simulink model "TrabControle"  (R2018b)
settings: Solver=VariableStepAuto  StartTime=0.0  StopTime=100  RelTol=1e-3
libraries: simulink x28
settings Model: Creator=Azeli  LastModifiedBy=Azeli

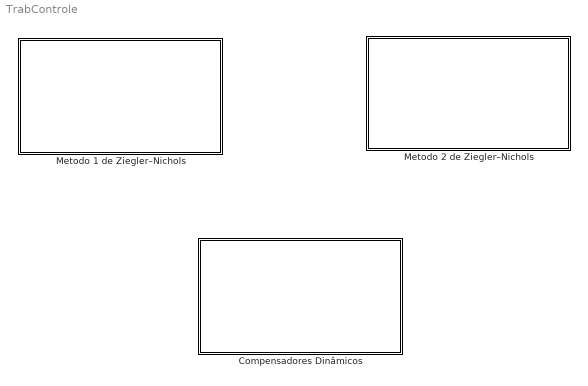
== system TrabControle ==
  Compensadores Dinâmicos : Subsystem
  "Metodo 1 de Ziegler–Nichols " : Subsystem
  "Metodo 2 de Ziegler–Nichols " : Subsystem

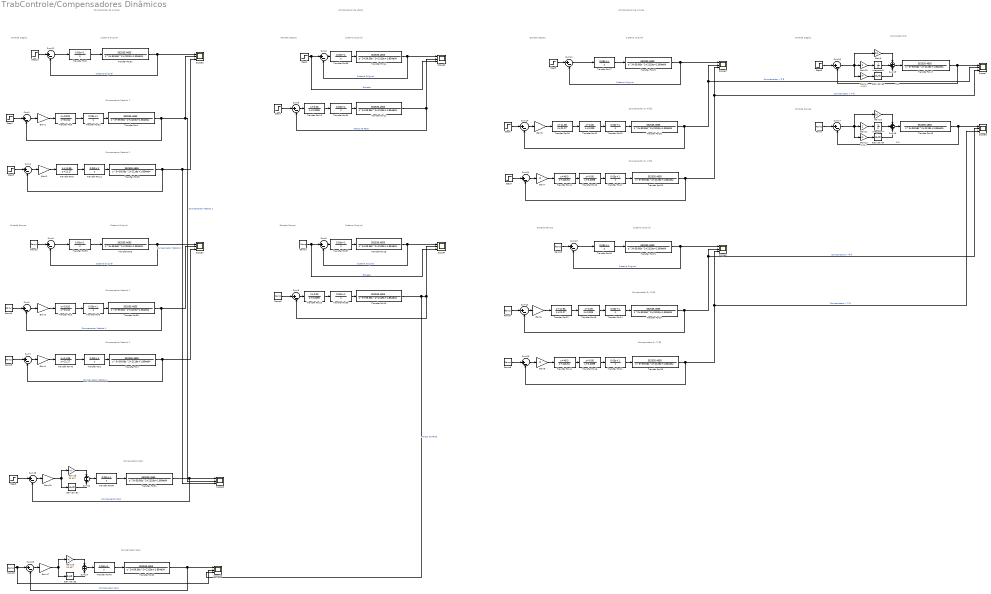
== system TrabControle/Compensadores Dinâmicos ==
  note: Compensador de Avanço
  note: Sistema Original
  note: Compensador Método 1
  note: Compensador Método 2
  note: Sistema Original
  note: Entrada Degrau
  note: Entrada Rampa
  note: Compensador de Atraso
  note: Sistema Original
  note: Sistema Original
  note: Entrada Rampa
  note: Entrada Degrau
  note: Compensador de Avanço
  note: Entrada Degrau
  note: Sistema Original
  note: Entrada Rampa
  note: Sistema Original
  note: Compensador Método 1
  note: Compensador Método 2
  note: Compensador $γ ≠ β$
  note: Compensador $γ = β$
  note: Compensador $γ ≠ β$
  note: Compensador $γ = β$
  note: Controlador PID
  note: Entrada Degrau
  note: Entrada Rampa
  note: Compensador Zero
  note: Compensador Zero
  Derivative{1..4} (4 alike) : Derivative
  Gain1 : Gain  Gain=1.6644
  Gain10 : Gain  Gain=0.1
  Gain11 : Gain  Gain=2
  Gain12 : Gain  Gain=0.004
  Gain13 : Gain  Gain=2
  Gain14 : Gain  Gain=0.004
  Gain15 : Gain  Gain=0.0290
  Gain16 : Gain  Gain=55.897
  Gain17 : Gain  Gain=0.0290
  Gain18 : Gain  Gain=55.897
  Gain{2,4..6} (4 alike) : Gain  Gain=1.3668
  Gain3 : Gain  Gain=1.6644
  Gain7 : Gain  Gain=8
  Gain8 : Gain  Gain=8
  Gain9 : Gain  Gain=0.1
  Integrator3 : Integrator
  Integrator4 : Integrator
  Ramp{,1..9} (10 alike) : simulink/Sources/Ramp  slope=1  start=0  InitialOutput=0
  Scope{1..10} (10 alike) : Scope  NumInputPorts=3
  Step{1..10} (10 alike) : Step  Time=0  After=10  SampleTime=0
  Sum{1..15,17..18,20..21,23} (20 alike) : Sum  Inputs=|+-
  Sum16 : Sum  Inputs=+++
  Sum19 : Sum  Inputs=+++
  Sum22 : Sum
  Sum24 : Sum
  Transfer Fcn{1,6,8,11,17,20..21,24,27,30,32,34..37,39,49..50} (18 alike) : TransferFcn  Numerator=[0.03 1]  Denominator=[1 0]
  Transfer Fcn{4..5,7,10,12,14,16,19,23,25..26,28..29,31,33,38,47..48,51..52} (20 alike) : TransferFcn  Numerator=[352535.4655]  Denominator=[1 59.56 2119 1.854e04]
  Transfer Fcn13 : TransferFcn  Numerator=[1 0.05]  Denominator=[1 0.0095]
  Transfer Fcn15 : TransferFcn  Numerator=[1 0.05]  Denominator=[1 0.0095]
  Transfer Fcn{9,18,22,40} (4 alike) : TransferFcn  Numerator=[1 11.96]  Denominator=[1 21.27]
  Transfer Fcn2 : TransferFcn  Numerator=[1 19.81]  Denominator=[1 31.54]
  Transfer Fcn3 : TransferFcn  Numerator=[1 19.81]  Denominator=[1 31.54]
  Transfer Fcn41 : TransferFcn  Numerator=[1 48.3]  Denominator=[1 246.91]
  Transfer Fcn42 : TransferFcn  Numerator=[1 0.06]  Denominator=[1 0.005]
  Transfer Fcn43 : TransferFcn  Numerator=[1 0.05]  Denominator=[1 0.0098]
  Transfer Fcn44 : TransferFcn  Numerator=[1 48.3]  Denominator=[1 246.91]
  Transfer Fcn45 : TransferFcn  Numerator=[1 0.06]  Denominator=[1 0.005]
  Transfer Fcn46 : TransferFcn  Numerator=[1 0.05]  Denominator=[1 0.0098]
  wires:
  Transfer Fcn4/1 -> Sum1/2, Scope9/2, Scope2/2  "Compensador Método 1"
  Step2/1 -> Sum1/1
  Step10/1 -> Sum21/1
  Sum21/1 -> Transfer Fcn8/1
  Transfer Fcn3/1 -> Transfer Fcn32/1
  Gain1/1 -> Transfer Fcn3/1
  Sum1/1 -> Gain1/1
  Transfer Fcn31/1 -> Sum21/2, Scope2/1  "Sistema Original"
  Transfer Fcn33/1 -> Sum4/2, Scope9/3, Scope2/3  "Compensador Método 2"
  Step4/1 -> Sum5/1
  Transfer Fcn12/1 -> Scope3/2, Sum5/2  "Atraso de Fase"
  Sum5/1 -> Transfer Fcn13/1
  Transfer Fcn14/1 -> Scope3/1, Sum6/2  "Sistema Original"
  Step1/1 -> Scope3/3, Sum6/1  "Entrada"
  Ramp2/1 -> Sum2/1
  Ramp5/1 -> Sum7/1
  Ramp6/1 -> Sum8/1
  Transfer Fcn8/1 -> Transfer Fcn31/1
  Transfer Fcn32/1 -> Transfer Fcn4/1
  Step3/1 -> Sum4/1
  Transfer Fcn9/1 -> Transfer Fcn11/1
  Sum4/1 -> Gain2/1
  Transfer Fcn11/1 -> Transfer Fcn33/1
  Gain2/1 -> Transfer Fcn9/1
  Transfer Fcn13/1 -> Transfer Fcn34/1
  Transfer Fcn34/1 -> Transfer Fcn12/1
  Sum6/1 -> Transfer Fcn35/1
  Transfer Fcn35/1 -> Transfer Fcn14/1
  Sum9/1 -> Transfer Fcn37/1
  Transfer Fcn37/1 -> Transfer Fcn16/1
  Sum8/1 -> Transfer Fcn15/1
  Ramp7/1 -> Scope4/3, Sum9/1  "Entrada"
  Transfer Fcn36/1 -> Transfer Fcn10/1
  Transfer Fcn15/1 -> Transfer Fcn36/1
  Transfer Fcn16/1 -> Scope4/1, Sum9/2  "Sistema Original"
  Transfer Fcn10/1 -> Scope10/3, Scope4/2, Sum8/2  "Atraso de Fase"
  Transfer Fcn1/1 -> Transfer Fcn7/1
  Transfer Fcn40/1 -> Transfer Fcn1/1
  Transfer Fcn6/1 -> Transfer Fcn38/1
  Transfer Fcn39/1 -> Transfer Fcn5/1
  Transfer Fcn5/1 -> Sum3/2, Scope1/1  "Sistema Original"
  Transfer Fcn2/1 -> Transfer Fcn6/1
  Gain3/1 -> Transfer Fcn2/1
  Sum2/1 -> Gain3/1
  Transfer Fcn7/1 -> Sum7/2, Scope1/3  "Compensador Método 2"
  Sum7/1 -> Gain4/1
  Sum3/1 -> Transfer Fcn39/1
  Transfer Fcn38/1 -> Sum2/2, Scope1/2  "Compensador Método 1"
  Ramp1/1 -> Sum3/1
  Gain7/1 -> Transfer Fcn41/1
  Transfer Fcn17/1 -> Transfer Fcn25/1
  Transfer Fcn20/1 -> Transfer Fcn26/1
  Step6/1 -> Sum10/1
  Transfer Fcn27/1 -> Transfer Fcn19/1
  Transfer Fcn19/1 -> Sum11/2, Scope5/1  "Sistema Original"
  Step7/1 -> Sum14/1
  Transfer Fcn25/1 -> Sum14/2, Scope7/3, Scope5/3  "Compensador γ = β"
  Sum14/1 -> Gain7/1
  Sum11/1 -> Transfer Fcn27/1
  Transfer Fcn26/1 -> Sum10/2, Scope5/2, Scope7/2  "Compensador γ ≠ β"
  Step5/1 -> Sum11/1
  Transfer Fcn42/1 -> Transfer Fcn20/1
  Transfer Fcn18/1 -> Transfer Fcn42/1
  Transfer Fcn41/1 -> Transfer Fcn43/1
  Transfer Fcn43/1 -> Transfer Fcn17/1
  Transfer Fcn44/1 -> Transfer Fcn46/1
  Transfer Fcn46/1 -> Transfer Fcn21/1
  Sum13/1 -> Transfer Fcn30/1
  Transfer Fcn29/1 -> Sum12/2, Scope8/2, Scope6/2  "Compensador γ ≠ β"
  Ramp4/1 -> Sum12/1
  Sum12/1 -> Gain6/1
  Transfer Fcn30/1 -> Transfer Fcn23/1
  Sum15/1 -> Gain8/1
  Transfer Fcn24/1 -> Transfer Fcn29/1
  Transfer Fcn21/1 -> Transfer Fcn28/1
  Transfer Fcn45/1 -> Transfer Fcn24/1
  Transfer Fcn28/1 -> Sum15/2, Scope8/3, Scope6/3  "Compensador γ = β"
  Ramp8/1 -> Sum15/1
  Gain8/1 -> Transfer Fcn44/1
  Transfer Fcn23/1 -> Sum13/2, Scope6/1  "Sistema Original"
  Ramp3/1 -> Sum13/1
  Gain4/1 -> Transfer Fcn40/1
  Gain5/1 -> Transfer Fcn18/1
  Sum10/1 -> Gain5/1
  Transfer Fcn22/1 -> Transfer Fcn45/1
  Gain6/1 -> Transfer Fcn22/1
  Gain9/1 -> Sum19/1
  Gain11/1 -> Integrator4/1
  Sum19/1 -> Transfer Fcn47/1
  Sum20/1 -> Gain9/1, Gain14/1, Gain13/1
  Integrator4/1 -> Sum16/2
  Gain13/1 -> Integrator3/1
  Derivative3/1 -> Sum19/3
  Integrator3/1 -> Sum19/2
  Gain10/1 -> Sum16/1
  Transfer Fcn47/1 -> Scope7/1, Sum20/2  "PID"
  Sum17/1 -> Gain10/1, Gain12/1, Gain11/1
  Step8/1 -> Sum20/1
  Transfer Fcn48/1 -> Scope8/1, Sum17/2  "PID"
  Sum16/1 -> Transfer Fcn48/1
  Gain14/1 -> Derivative3/1
  Ramp/1 -> Sum17/1
  Derivative4/1 -> Sum16/3
  Gain12/1 -> Derivative4/1
  Transfer Fcn50/1 -> Transfer Fcn51/1
  Sum18/1 -> Gain15/1
  Gain15/1 -> Derivative1/1, Gain16/1
  Sum22/1 -> Transfer Fcn50/1
  Step9/1 -> Sum18/1
  Transfer Fcn51/1 -> Scope9/1, Sum18/2  "Compensador Zero"
  Gain16/1 -> Sum22/1
  Derivative1/1 -> Sum22/2
  Transfer Fcn52/1 -> Scope10/1, Sum23/2  "Compensador Zero"
  Ramp9/1 -> Scope10/2, Sum23/1
  Sum23/1 -> Gain17/1
  Transfer Fcn49/1 -> Transfer Fcn52/1
  Gain18/1 -> Sum24/1
  Sum24/1 -> Transfer Fcn49/1
  Gain17/1 -> Derivative2/1, Gain18/1
  Derivative2/1 -> Sum24/2

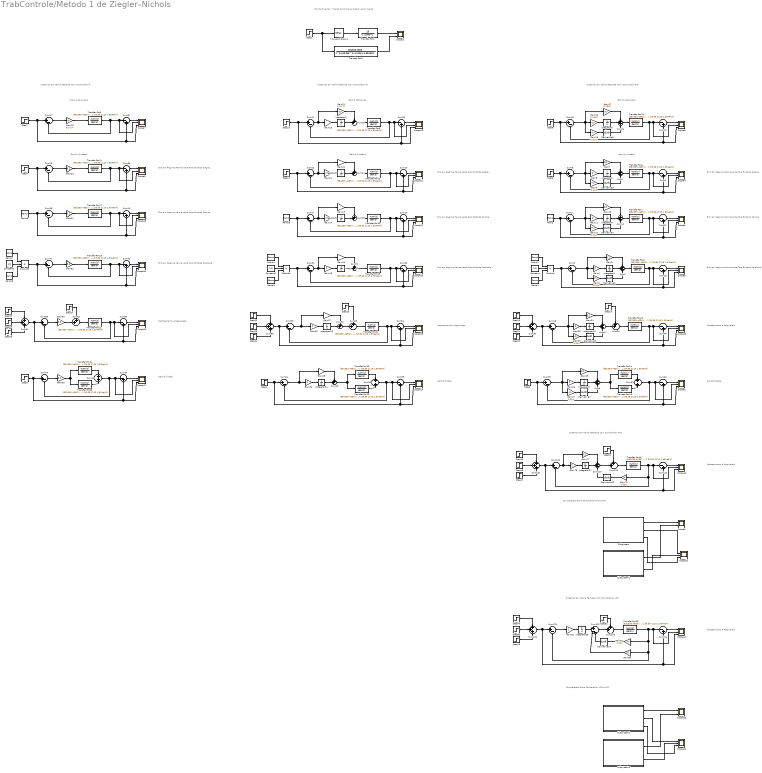
== system TrabControle/Metodo 1 de Ziegler–Nichols  ==
  note: Ganho Calculado
  note: Planta Original x Planta de Primeira Ordem Aproximada
  note: Sistemas em Malha Fechada Com Controlador P
  note: Ganho Ajustado
  note: Erro em Regime Permanente Para Entrada Degrau
  note: Erro em Regime Permanente Para Entrada Rampa
  note: Erro em Regime Permanente Para Entrada Parábola
  note: Rastreamento e Regulação
  note: Sensibilidade
  note: Erro em Regime Permanente Para Entrada Degrau
  note: Erro em Regime Permanente Para Entrada Parábola
  note: Sensibilidade
  note: Erro em Regime Permanente Para Entrada Rampa
  note: Rastreamento e Regulação
  note: Ganho Calculado
  note: Sistemas em Malha Fechada Com Controlador PI
  note: Ganho Ajustado
  note: Sensibilidade
  note: Erro em Regime Permanente Para Entrada Degrau
  note: Rastreamento e Regulação
  note: Erro em Regime Permanente Para Entrada Rampa
  note: Erro em Regime Permanente Para Entrada Parábola
  note: Ganho Calculado
  note: Sistemas em Malha Fechada Com Controlador PID
  note: Sistemas em Malha Fechada Com Controlador PI-D
  note: Sistemas em Malha Fechada Com Controlador I-PD
  note: Rastreamento e Regulação
  note: Rastreamento e Regulação
  note: Ganho Ajustado
  note: Comparação Entre Controlador PI-D e PID
  note: Comparação Entre Controlador I-PD e PID
  Constant : Constant  Value=1/2
  Constant1 : Constant  Value=1/2
  Constant2 : Constant  Value=1/2
  Derivative{1,3..7,13..14} (8 alike) : Derivative
  Gain{3,7,10,20,25,31..34,39,77,80} (12 alike) : Gain  Gain=0.1
  Gain{4,8,11,26,35,78,81} (7 alike) : Gain  Gain=2
  Gain{5,9,12,27,36,79,82} (7 alike) : Gain  Gain=0.004
  Gain{13,15,22,29,37} (5 alike) : Gain  Gain=0.06
  Gain{14,24,28,30,38} (5 alike) : Gain
  Gain16 : Gain  Gain=0.2414
  Gain17 : Gain  Gain=0.2897
  Gain18 : Gain  Gain=5.1548
  Gain19 : Gain  Gain=0.0041
  Gain21 : Gain  Gain=0.2173
  Gain23 : Gain  Gain=2.32
  Integrator{1,3..13,27..28} (14 alike) : Integrator
  Product : Product  Inputs=3
  Product1 : Product  Inputs=3
  Product2 : Product  Inputs=3
  Ramp{,1..8} (9 alike) : simulink/Sources/Ramp  slope=1  start=0  InitialOutput=0
  Scope1 : Scope  NumInputPorts=2
  Scope{2,4..22,40..41} (22 alike) : Scope  NumInputPorts=3
  Scope23 : Scope  NumInputPorts=2
  Scope3 : Scope  NumInputPorts=2
  Step1 : Step  Time=0  SampleTime=0
  Step{2,4..11,18,22,26,43..44} (14 alike) : Step  Time=0  After=10  SampleTime=0
  Step{19,23,27,51..52} (5 alike) : Step  Time=8  After=2  SampleTime=0
  Step{20,24,28,47,49} (5 alike) : Step  Time=6  After=5  SampleTime=0
  Step{21,25,29,48,50} (5 alike) : Step  Time=3  After=-10  SampleTime=0
  Subsystem : Subsystem
  Subsystem1 : Subsystem
  Subsystem2 : Subsystem
  Subsystem3 : Subsystem
  Sum{2,6..7,10,16,47,51,56,61,131..132} (11 alike) : Sum  Inputs=+++
  Sum{3,8,11,17..18,20..22,25,27,31,34,39,41,44,48,53,58,120,123} (20 alike) : Sum  Inputs=|+-
  Sum119 : Sum  Inputs=++-
  Sum{9,12..15,19,26,29..30,35,37..38,40,42,45,49,54,59,121,124} (20 alike) : Sum  Inputs=|-+
  Sum122 : Sum  Inputs=|+|--
  Sum{23..24,28,32,43,50,52,55,60,133..134} (11 alike) : Sum  Inputs=++|
  Sum33 : Sum  Inputs=+|+
  Sum36 : Sum  Inputs=+|+
  Sum46 : Sum  Inputs=+|+
  Transfer Fcn1 : TransferFcn  Numerator=[19]  Denominator=[0.1289 1]
  Transfer Fcn{2,5..25,48..49} (24 alike) : TransferFcn  Numerator=[352535.4655]  Denominator=[1 59.56 2119 1.854e04]
  Transport Delay1 : TransportDelay  DelayTime=0.0281
  wires:
  Sum31/1 -> Gain15/1, Gain28/1
  Gain4/1 -> Integrator1/1
  Transfer Fcn1/1 -> Scope1/1
  Ramp3/1 -> Scope12/3, Sum14/2, Sum27/1
  Step9/1 -> Sum38/2, Scope9/3, Sum20/1
  Transfer Fcn48/1 -> Sum120/2, Gain79/1, Scope40/2, Sum121/1
  Transfer Fcn8/1 -> Scope10/2, Sum29/1, Sum21/2
  Transfer Fcn24/1 -> Sum46/1
  Product/1 -> Sum3/1, Sum15/2, Scope6/3
  Sum45/1 -> Scope17/1
  Gain27/1 -> Derivative7/1
  Derivative6/1 -> Sum16/3
  Gain32/1 -> Transfer Fcn18/1
  Transfer Fcn10/1 -> Scope8/2, Sum19/1, Sum18/2
  Sum19/1 -> Scope8/1
  Integrator5/1 -> Sum28/2
  Step7/1 -> Sum37/2, Scope7/3, Sum17/1
  Sum38/1 -> Scope9/1
  Sum56/1 -> Sum54/2, Scope19/3, Sum53/1
  Step1/1 -> Transfer Fcn5/1, Transport Delay1/1
  Ramp5/1 -> Product1/3
  Transfer Fcn21/1 -> Scope19/2, Sum54/1, Sum53/2
  Step11/1 -> Scope11/3, Sum13/2, Sum22/1
  Sum7/1 -> Transfer Fcn6/1
  Derivative3/1 -> Sum7/3
  Gain26/1 -> Integrator9/1
  Gain36/1 -> Derivative5/1
  Step8/1 -> Sum19/2, Scope8/3, Sum18/1
  Transfer Fcn6/1 -> Scope4/2, Sum9/1, Sum8/2
  Transport Delay1/1 -> Transfer Fcn1/1
  Step49/1 -> Sum132/3
  Sum3/1 -> Gain3/1, Gain5/1, Gain4/1
  Derivative4/1 -> Sum10/3
  Ramp1/1 -> Product/1
  Ramp2/1 -> Product/3
  Sum21/1 -> Gain21/1, Gain23/1
  Transfer Fcn5/1 -> Scope1/2
  Step6/1 -> Sum9/2, Scope4/3, Sum8/1
  Sum39/1 -> Gain31/1
  Gain25/1 -> Sum6/1
  Step2/1 -> Sum26/2, Scope2/3, Sum25/1
  Integrator1/1 -> Sum2/2
  Step43/1 -> Sum131/1
  Gain9/1 -> Derivative3/1
  Product2/1 -> Sum42/2, Scope16/3, Sum41/1
  Gain8/1 -> Integrator3/1
  Gain11/1 -> Integrator4/1
  Transfer Fcn7/1 -> Scope5/2, Sum12/1, Sum11/2
  Sum50/1 -> Transfer Fcn20/1
  Integrator6/1 -> Sum16/2
  Sum27/1 -> Gain13/1, Gain14/1
  Sum47/1 -> Sum50/2
  Sum2/1 -> Transfer Fcn2/1
  Integrator12/1 -> Sum47/2
  Gain12/1 -> Derivative4/1
  Transfer Fcn17/1 -> Sum39/2, Scope15/2, Sum40/1
  Step21/1 -> Sum51/2
  Sum16/1 -> Transfer Fcn10/1
  Sum33/1 -> Scope2/2, Sum26/1, Sum25/2
  Sum54/1 -> Scope19/1
  Sum10/1 -> Transfer Fcn7/1
  Sum17/1 -> Gain16/1
  Sum46/1 -> Scope17/2, Sum45/1, Sum44/2
  Step24/1 -> Sum56/3
  Gain17/1 -> Sum16/1
  Gain82/1 -> Derivative14/1
  Gain24/1 -> Integrator8/1
  Transfer Fcn12/1 -> Scope11/2, Sum13/1, Sum22/2
  Sum32/1 -> Transfer Fcn15/1
  Transfer Fcn49/1 -> Sum123/2, Gain80/1, Gain82/1, Scope41/2, Sum124/1
  Sum15/1 -> Scope6/1
  Transfer Fcn20/1 -> Scope18/2, Sum49/1, Sum48/2
  Sum24/1 -> Transfer Fcn12/1
  Sum133/1 -> Transfer Fcn48/1
  Transfer Fcn11/1 -> Sum20/2, Scope9/2, Sum38/1
  Transfer Fcn18/1 -> Sum41/2, Scope16/2, Sum42/1
  Ramp/1 -> Sum12/2, Scope5/3, Sum11/1
  Gain16/1 -> Transfer Fcn9/1
  Sum53/1 -> Gain38/1, Gain37/1
  Gain22/1 -> Sum24/1
  Sum30/1 -> Scope13/1
  Sum22/1 -> Gain22/1, Gain24/1
  Transfer Fcn9/1 -> Sum17/2, Scope7/2, Sum37/1
  Sum25/1 -> Gain25/1, Gain27/1, Gain26/1
  Sum23/1 -> Transfer Fcn8/1
  Gain15/1 -> Sum32/1
  Sum11/1 -> Gain10/1, Gain12/1, Gain11/1
  Step28/1 -> Sum61/3
  Sum37/1 -> Scope7/1
  Transfer Fcn14/1 -> Sum33/1
  Ramp4/1 -> Product1/1
  Transfer Fcn22/1 -> Scope20/2, Sum59/1, Sum58/2
  Ramp6/1 -> Sum40/2, Scope15/3, Sum39/1
  Sum18/1 -> Gain17/1, Gain19/1, Gain18/1
  Gain33/1 -> Transfer Fcn25/1, Transfer Fcn24/1
  Step4/1 -> Sum35/2, Scope14/3, Sum34/1
  Constant1/1 -> Product1/2
  Sum8/1 -> Gain7/1, Gain9/1, Gain8/1
  Step10/1 -> Sum29/2, Scope10/3, Sum21/1
  Sum55/1 -> Transfer Fcn21/1
  Step5/1 -> Sum45/2, Scope17/3, Sum44/1
  Product1/1 -> Scope13/3, Sum30/2, Sum31/1
  Integrator7/1 -> Sum23/2
  Gain19/1 -> Derivative6/1
  Gain23/1 -> Integrator7/1
  Sum6/1 -> Transfer Fcn16/1, Transfer Fcn14/1
  Gain21/1 -> Sum23/1
  Sum61/1 -> Sum59/2, Scope20/3, Sum58/1
  Sum28/1 -> Transfer Fcn13/1
  Integrator3/1 -> Sum7/2
  Integrator4/1 -> Sum10/2
  Sum14/1 -> Scope12/1
  Derivative1/1 -> Sum2/3
  Sum36/1 -> Scope14/2, Sum35/1, Sum34/2
  Integrator28/1 -> Sum122/1
  Sum40/1 -> Scope15/1
  Sum20/1 -> Gain20/1
  Gain28/1 -> Integrator10/1
  Sum12/1 -> Scope5/1
  Step18/1 -> Sum51/1
  Sum43/1 -> Transfer Fcn23/1, Transfer Fcn19/1
  Step48/1 -> Sum131/2
  Gain80/1 -> Sum122/2
  Sum9/1 -> Scope4/1
  Sum26/1 -> Scope2/1
  Gain38/1 -> Integrator13/1
  Constant2/1 -> Product2/2
  Transfer Fcn19/1 -> Sum36/1
  Gain30/1 -> Integrator11/1
  Gain37/1 -> Sum52/1
  Sum49/1 -> Scope18/1
  Sum60/1 -> Transfer Fcn22/1
  Sum134/1 -> Transfer Fcn49/1
  Gain39/1 -> Sum60/2
  Gain29/1 -> Sum43/1
  Sum59/1 -> Scope20/1
  Step20/1 -> Sum51/3
  Sum44/1 -> Gain33/1
  Transfer Fcn16/1 -> Sum33/2
  Ramp8/1 -> Product2/3
  Derivative5/1 -> Sum47/3
  Sum13/1 -> Scope11/1
  Sum58/1 -> Gain39/1
  Transfer Fcn13/1 -> Scope12/2, Sum14/1, Sum27/2
  Step22/1 -> Sum56/1
  Sum51/1 -> Sum49/2, Scope18/3, Sum48/1
  Integrator11/1 -> Sum43/2
  Ramp7/1 -> Product2/1
  Gain20/1 -> Transfer Fcn11/1
  Gain13/1 -> Sum28/1
  Transfer Fcn2/1 -> Sum15/1, Scope6/2, Sum3/2
  Sum48/1 -> Gain34/1, Gain36/1, Gain35/1
  Sum42/1 -> Scope16/1
  Transfer Fcn15/1 -> Scope13/2, Sum30/1, Sum31/2
  Gain31/1 -> Transfer Fcn17/1
  Integrator9/1 -> Sum6/2
  Sum124/1 -> Scope41/1
  Sum132/1 -> Sum124/2, Scope41/3, Sum123/1
  Step51/1 -> Sum133/1
  Integrator8/1 -> Sum24/2
  Sum29/1 -> Scope10/1
  Sum52/1 -> Sum55/2
  Sum131/1 -> Sum121/2, Scope40/3, Sum120/1
  Integrator27/1 -> Sum119/2
  Step19/1 -> Sum50/1
  Integrator13/1 -> Sum52/2
  Step50/1 -> Sum132/2
  Step23/1 -> Sum55/1
  Gain10/1 -> Sum10/1
  Gain78/1 -> Integrator27/1
  Sum120/1 -> Gain78/1, Gain77/1
  Step27/1 -> Sum60/1
  Integrator10/1 -> Sum32/2
  Derivative14/1 -> Sum122/3
  Step29/1 -> Sum61/2
  Step26/1 -> Sum61/1
  Gain14/1 -> Integrator5/1
  Sum34/1 -> Gain29/1, Gain30/1
  Gain77/1 -> Sum119/1
  Gain5/1 -> Derivative1/1
  Transfer Fcn25/1 -> Sum46/2
  Constant/1 -> Product/2
  Gain18/1 -> Integrator6/1
  Gain3/1 -> Sum2/1
  Derivative13/1 -> Sum119/3
  Transfer Fcn23/1 -> Sum36/2
  Sum121/1 -> Scope40/1
  Gain81/1 -> Integrator28/1
  Gain79/1 -> Derivative13/1
  Gain7/1 -> Sum7/1
  Step25/1 -> Sum56/2
  Gain34/1 -> Sum47/1
  Sum35/1 -> Scope14/1
  Sum119/1 -> Sum133/2
  Derivative7/1 -> Sum6/3
  Sum122/1 -> Sum134/2
  Step52/1 -> Sum134/1
  Sum41/1 -> Gain32/1
  Sum123/1 -> Gain81/1
  Gain35/1 -> Integrator12/1
  Step44/1 -> Sum132/1
  Step47/1 -> Sum131/3
  Subsystem/1(Erro PID) -> Scope3/1  "Erro PID"
  Subsystem1/1(Erro PI-D) -> Scope3/2  "Erro PI-D"
  Subsystem/2(Saída PID) -> Scope21/1  "Saída PID"
  Subsystem1/2(Saída PI-D) -> Scope21/2  "Saída PI-D"
  Subsystem/3(Entrada PID) -> Scope21/3  "Entrada"
  Subsystem2/3(Entrada I-PD) -> Scope22/3  "Entrada"
  Subsystem3/1(Erro PID) -> Scope23/2  "Erro PID"
  Subsystem2/1(Erro I-PD) -> Scope23/1  "Erro I-PD"
  Subsystem2/2(Saída I-PD) -> Scope22/1  "Saida I-PD"
  Subsystem3/2(Saída PID) -> Scope22/2  "Saída PID"

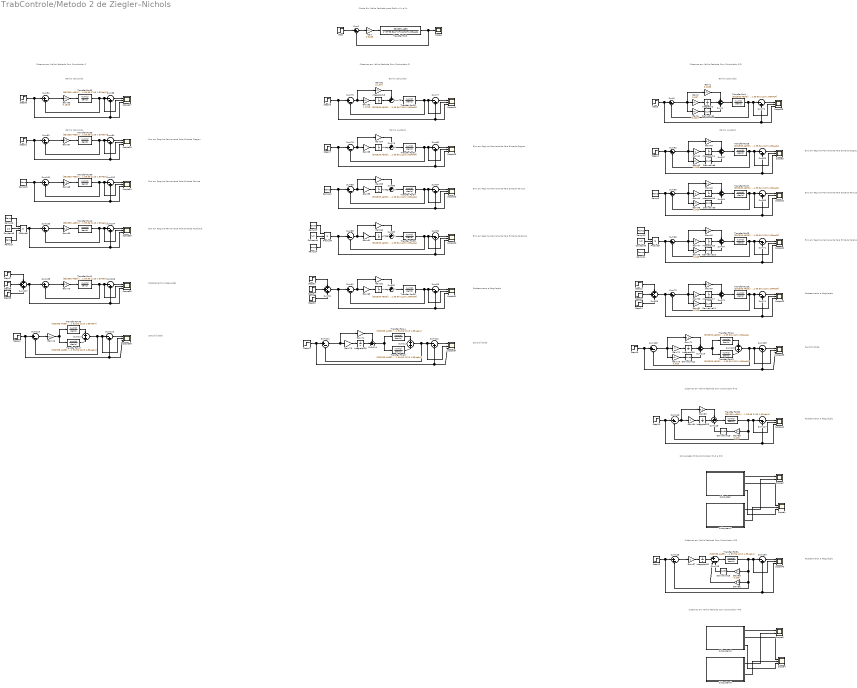
== system TrabControle/Metodo 2 de Ziegler–Nichols  ==
  note: Planta Em Malha Fechada para Definir Ku e Pu
  note: Ganho Calculado
  note: Sistemas em Malha Fechada Com Controlador PI
  note: Ganho Ajustado
  note: Erro em Regime Permanente Para Entrada Degrau
  note: Erro em Regime Permanente Para Entrada Parábola
  note: Sensibilidade
  note: Erro em Regime Permanente Para Entrada Rampa
  note: Rastreamento e Regulação
  note: Ganho Calculado
  note: Sistemas em Malha Fechada Com Controlador P
  note: Ganho Calculado
  note: Erro em Regime Permanente Para Entrada Parábola
  note: Erro em Regime Permanente Para Entrada Rampa
  note: Erro em Regime Permanente Para Entrada Degrau
  note: Sensibilidade
  note: Rastreamento e Regulação
  note: Erro em Regime Permanente Para Entrada Parábola
  note: Erro em Regime Permanente Para Entrada Rampa
  note: Erro em Regime Permanente Para Entrada Degrau
  note: Sensibilidade
  note: Rastreamento e Regulação
  note: Sistemas em Malha Fechada Com Controlador PID
  note: Ganho Calculado
  note: Ganho Ajustado
  note: Sistemas em Malha Fechada Com Controlador PI-D
  note: Rastreamento e Regulação
  note: Rastreamento e Regulação
  note: Sistemas em Malha Fechada Com Controlador I-PD
  note: Comparação Entre Controlador PI-D e PID
  note: Sistemas em Malha Fechada Com Controlador I-PD
  Constant3 : Constant  Value=1/2
  Constant4 : Constant  Value=1/2
  Constant5 : Constant  Value=1/2
  Derivative{2,8..12,15..16} (8 alike) : Derivative
  Gain : Gain  Gain=0.3055
  Gain1 : Gain  Gain=0.1833
  Gain2 : Gain  Gain=2.657
  Gain{40,43,46,49,57,68..71,76,83,86} (12 alike) : Gain  Gain=0.1
  Gain{41,44,47,50,72,84,87} (7 alike) : Gain  Gain=2
  Gain{42,45,48,51,73,85,88} (7 alike) : Gain  Gain=0.005
  Gain52 : Gain  Gain=0.1375
  Gain53 : Gain  Gain=1.1948
  Gain{54,58,60,62,74} (5 alike) : Gain  Gain=0.05
  Gain{55,59,61,63,75} (5 alike) : Gain  Gain=0.85
  Gain56 : Gain  Gain=0.1528
  Gain6 : Gain  Gain=0.0037
  Integrator{2,14..22,25..26,29..30} (14 alike) : Integrator
  Product3 : Product  Inputs=3
  Product4 : Product  Inputs=3
  Product5 : Product  Inputs=3
  Ramp{9..17} (9 alike) : simulink/Sources/Ramp  slope=1  start=0  InitialOutput=0
  Scope : Scope
  Scope{1,3..4,21..31,34..39,42..43} (22 alike) : Scope  NumInputPorts=3
  Scope2 : Scope  NumInputPorts=2
  Scope5 : Scope  NumInputPorts=2
  Step : Step  Time=0  SampleTime=0
  Step{3,12..13,16..17,30..32,37,40..42,45..46} (14 alike) : Step  Time=0  After=10  SampleTime=0
  Step14 : Step  Time=6  After=5  SampleTime=0
  Step15 : Step  Time=3  After=-10  SampleTime=0
  Step33 : Step  Time=6  After=5  SampleTime=0
  Step34 : Step  Time=3  After=-10  SampleTime=0
  Step38 : Step  Time=6  After=5  SampleTime=0
  Step39 : Step  Time=3  After=-10  SampleTime=0
  Subsystem : Subsystem
  Subsystem1 : Subsystem
  Subsystem2 : Subsystem
  Subsystem3 : Subsystem
  Sum{1,5,62,65,68,73,75,78,81..82,85,88,91,101,103,105,108,111,115,126,129} (21 alike) : Sum  Inputs=|+-
  Sum{63,66,70..71,74,77,80,83..84,87,90,93,102,104,106,109,112,116,127,130} (20 alike) : Sum  Inputs=|-+
  Sum{4,57,64,67,69,72,94,107,118} (9 alike) : Sum  Inputs=+++
  Sum110 : Sum  Inputs=+|+
  Sum113 : Sum  Inputs=+|+
  Sum{76,79,86,89,92,114} (6 alike) : Sum  Inputs=++|
  Sum117 : Sum  Inputs=+|+
  Sum125 : Sum  Inputs=++-
  Sum128 : Sum  Inputs=|+|--
  Transfer Fcn{3..4,26..36,39..47,50..51} (24 alike) : TransferFcn  Numerator=[352535.4655]  Denominator=[1 59.56 2119 1.854e04]
  wires:
  Transfer Fcn3/1 -> Scope/1, Sum1/2
  Transfer Fcn36/1 -> Scope31/2, Sum93/1, Sum91/2
  Gain52/1 -> Sum76/1
  Product5/1 -> Sum103/1, Sum104/2, Scope35/3
  Transfer Fcn41/1 -> Scope36/2, Sum106/1, Sum105/2
  Sum79/1 -> Transfer Fcn31/1
  Integrator21/1 -> Sum89/2
  Sum68/1 -> Gain46/1, Gain48/1, Gain47/1
  Sum5/1 -> Gain1/1, Gain6/1, Gain2/1
  Sum87/1 -> Scope29/1
  Derivative9/1 -> Sum64/3
  Transfer Fcn33/1 -> Scope28/2, Sum84/1, Sum82/2
  Gain71/1 -> Sum118/1
  Step/1 -> Sum1/1
  Derivative10/1 -> Sum67/3
  Sum70/1 -> Scope25/1
  Ramp15/1 -> Sum102/2, Scope34/3, Sum101/1
  Transfer Fcn4/1 -> Sum70/1, Scope25/2, Sum5/2
  Gain84/1 -> Integrator29/1
  Step46/1 -> Sum130/2, Scope43/3, Sum129/1
  Transfer Fcn51/1 -> Sum129/2, Gain86/1, Gain88/1, Scope43/2, Sum130/1
  Sum65/1 -> Gain43/1, Gain45/1, Gain44/1
  Transfer Fcn30/1 -> Scope24/2, Sum77/1, Sum75/2
  Sum85/1 -> Gain58/1, Gain59/1
  Sum69/1 -> Scope23/3, Sum74/2, Sum73/1
  Sum125/1 -> Transfer Fcn50/1
  Ramp12/1 -> Sum87/2, Scope29/3, Sum85/1
  Gain76/1 -> Transfer Fcn47/1, Transfer Fcn46/1
  Step33/1 -> Sum94/3
  Sum64/1 -> Transfer Fcn27/1
  Transfer Fcn45/1 -> Sum113/2
  Transfer Fcn29/1 -> Sum74/1, Scope23/2, Sum73/2
  Step41/1 -> Sum112/2, Scope37/3, Sum111/1
  Sum113/1 -> Scope37/2, Sum112/1, Sum111/2
  Transfer Fcn26/1 -> Sum63/1, Scope3/2, Sum62/2
  Sum57/1 -> Transfer Fcn26/1
  Step17/1 -> Sum80/2, Scope26/3, Sum78/1
  Sum107/1 -> Sum105/1, Sum106/2, Scope36/3
  Ramp9/1 -> Scope21/3, Sum66/2, Sum65/1
  Sum83/1 -> Scope27/1
  Transfer Fcn31/1 -> Scope26/2, Sum80/1, Sum78/2
  Sum90/1 -> Scope30/1
  Gain56/1 -> Transfer Fcn32/1
  Integrator22/1 -> Sum92/2
  Transfer Fcn50/1 -> Sum126/2, Gain85/1, Scope42/2, Sum127/1
  Step15/1 -> Sum69/2
  Gain44/1 -> Integrator15/1
  Integrator2/1 -> Sum4/2
  Integrator26/1 -> Sum118/2
  Gain50/1 -> Integrator17/1
  Sum93/1 -> Scope31/1
  Transfer Fcn43/1 -> Sum110/2
  Step16/1 -> Sum77/2, Scope24/3, Sum75/1
  Transfer Fcn34/1 -> Scope29/2, Sum87/1, Sum85/2
  Gain45/1 -> Derivative9/1
  Ramp14/1 -> Product4/3
  Step13/1 -> Sum69/1
  Ramp13/1 -> Product4/1
  Gain86/1 -> Sum128/2
  Integrator18/1 -> Sum76/2
  Sum1/1 -> Gain/1
  Transfer Fcn28/1 -> Sum71/1, Scope22/2, Sum68/2
  Sum63/1 -> Scope3/1
  Sum84/1 -> Scope28/1
  Step31/1 -> Sum84/2, Scope28/3, Sum82/1
  Product4/1 -> Sum90/2, Scope30/3, Sum88/1
  Gain40/1 -> Sum57/1
  Sum91/1 -> Gain62/1, Gain63/1
  Gain62/1 -> Sum92/1
  Sum66/1 -> Scope21/1
  Constant4/1 -> Product4/2
  Integrator19/1 -> Sum79/2
  Derivative12/1 -> Sum118/3
  Sum101/1 -> Gain68/1
  Gain58/1 -> Sum86/1
  Integrator15/1 -> Sum64/2
  Transfer Fcn32/1 -> Scope27/2, Sum83/1, Sum81/2
  Sum114/1 -> Transfer Fcn45/1, Transfer Fcn44/1
  Sum82/1 -> Gain57/1
  Gain59/1 -> Integrator20/1
  Sum110/1 -> Scope39/2, Sum109/1, Sum108/2
  Gain47/1 -> Integrator16/1
  Derivative11/1 -> Sum72/3
  Product3/1 -> Scope22/3, Sum71/2, Sum68/1
  Step30/1 -> Sum83/2, Scope27/3, Sum81/1
  Step45/1 -> Sum127/2, Scope42/3, Sum126/1
  Step12/1 -> Scope3/3, Sum63/2, Sum62/1
  Transfer Fcn27/1 -> Sum66/1, Scope21/2, Sum65/2
  Gain87/1 -> Integrator30/1
  Gain43/1 -> Sum64/1
  Sum108/1 -> Gain71/1, Gain73/1, Gain72/1
  Gain48/1 -> Derivative10/1
  Integrator14/1 -> Sum57/2
  Step3/1 -> Scope25/3, Sum70/2, Sum5/1
  Sum109/1 -> Scope39/1
  Ramp11/1 -> Product3/3
  Sum117/1 -> Scope38/2, Sum116/1, Sum115/2
  Gain42/1 -> Derivative8/1
  Gain74/1 -> Sum114/1
  Derivative2/1 -> Sum4/3
  Step42/1 -> Sum116/2, Scope38/3, Sum115/1
  Sum94/1 -> Sum93/2, Scope31/3, Sum91/1
  Sum105/1 -> Gain70/1
  Gain/1 -> Transfer Fcn3/1
  Transfer Fcn40/1 -> Scope35/2, Sum104/1, Sum103/2
  Constant5/1 -> Product5/2
  Step32/1 -> Sum94/1
  Transfer Fcn46/1 -> Sum117/1
  Sum81/1 -> Gain56/1
  Transfer Fcn47/1 -> Sum117/2
  Integrator30/1 -> Sum128/1
  Sum74/1 -> Scope23/1
  Constant3/1 -> Product3/2
  Sum103/1 -> Gain69/1
  Gain63/1 -> Integrator22/1
  Transfer Fcn39/1 -> Scope34/2, Sum102/1, Sum101/2
  Sum116/1 -> Scope38/1
  Sum102/1 -> Scope34/1
  Sum118/1 -> Transfer Fcn43/1, Transfer Fcn42/1
  Transfer Fcn42/1 -> Sum110/1
  Sum128/1 -> Transfer Fcn51/1
  Gain60/1 -> Sum89/1
  Sum76/1 -> Transfer Fcn30/1
  Gain70/1 -> Transfer Fcn41/1
  Sum77/1 -> Scope24/1
  Step40/1 -> Scope39/3, Sum109/2, Sum108/1
  Transfer Fcn35/1 -> Scope30/2, Sum90/1, Sum88/2
  Sum111/1 -> Gain74/1, Gain75/1
  Sum88/1 -> Gain60/1, Gain61/1
  Sum104/1 -> Scope35/1
  Gain46/1 -> Sum67/1
  Gain2/1 -> Integrator2/1
  Sum75/1 -> Gain52/1, Gain53/1
  Sum115/1 -> Gain76/1
  Sum126/1 -> Gain84/1, Gain83/1
  Sum67/1 -> Transfer Fcn28/1
  Sum78/1 -> Gain54/1, Gain55/1
  Step39/1 -> Sum107/2
  Gain54/1 -> Sum79/1
  Derivative15/1 -> Sum125/3
  Derivative8/1 -> Sum57/3
  Gain72/1 -> Integrator26/1
  Gain75/1 -> Integrator25/1
  Ramp17/1 -> Product5/3
  Sum71/1 -> Scope22/1
  Gain88/1 -> Derivative16/1
  Sum129/1 -> Gain87/1
  Gain6/1 -> Derivative2/1
  Integrator29/1 -> Sum125/2
  Gain68/1 -> Transfer Fcn39/1
  Integrator17/1 -> Sum72/2
  Gain73/1 -> Derivative12/1
  Integrator25/1 -> Sum114/2
  Step34/1 -> Sum94/2
  Integrator16/1 -> Sum67/2
  Ramp16/1 -> Product5/1
  Ramp10/1 -> Product3/1
  Sum73/1 -> Gain49/1, Gain51/1, Gain50/1
  Sum62/1 -> Gain40/1, Gain42/1, Gain41/1
  Step37/1 -> Sum107/1
  Gain55/1 -> Integrator19/1
  Derivative16/1 -> Sum128/3
  Sum80/1 -> Scope26/1
  Gain49/1 -> Sum72/1
  Gain69/1 -> Transfer Fcn40/1
  Sum92/1 -> Transfer Fcn36/1
  Gain83/1 -> Sum125/1
  Sum127/1 -> Scope42/1
  Gain51/1 -> Derivative11/1
  Sum112/1 -> Scope37/1
  Gain53/1 -> Integrator18/1
  Sum106/1 -> Scope36/1
  Gain57/1 -> Transfer Fcn33/1
  Gain41/1 -> Integrator14/1
  Gain1/1 -> Sum4/1
  Integrator20/1 -> Sum86/2
  Sum72/1 -> Transfer Fcn29/1
  Gain85/1 -> Derivative15/1
  Step14/1 -> Sum69/3
  Sum86/1 -> Transfer Fcn34/1
  Transfer Fcn44/1 -> Sum113/1
  Gain61/1 -> Integrator21/1
  Step38/1 -> Sum107/3
  Sum4/1 -> Transfer Fcn4/1
  Sum89/1 -> Transfer Fcn35/1
  Sum130/1 -> Scope43/1
  Subsystem1/2(Saída PI-D) -> Scope1/2  "Saída PI-D"
  Subsystem/3(Entrada PID) -> Scope1/3  "Entrada"
  Subsystem1/1(Erro PI-D) -> Scope2/2  "Erro PI-D"
  Subsystem/1(Erro PID) -> Scope2/1  "Erro PID"
  Subsystem/2(Saída PID) -> Scope1/1  "Saída PID"
  Subsystem2/2(Saída PID) -> Scope4/1  "Saída PID"
  Subsystem2/3(Entrada PID) -> Scope4/3  "Entrada"
  Subsystem3/2(Saída I-PD) -> Scope4/2  "Saída I-PD"
  Subsystem3/1(Erro I-PD) -> Scope5/2  "Erro I-PD"
  Subsystem2/1(Erro PID) -> Scope5/1  "Erro PID"

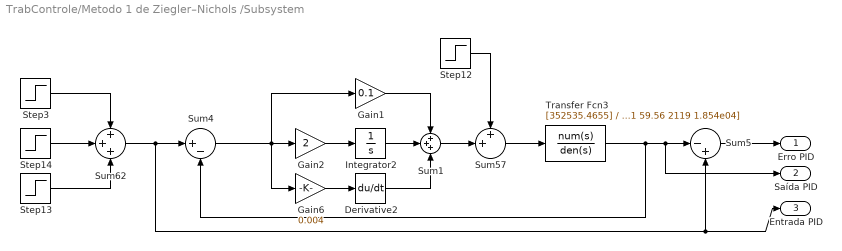
== system TrabControle/Metodo 1 de Ziegler–Nichols /Subsystem ==
  Derivative2 : Derivative
  Gain1 : Gain  Gain=0.1
  Gain2 : Gain  Gain=2
  Gain6 : Gain  Gain=0.004
  Integrator2 : Integrator
  Step12 : Step  Time=8  After=2  SampleTime=0
  Step13 : Step  Time=6  After=5  SampleTime=0
  Step14 : Step  Time=3  After=-10  SampleTime=0
  Step3 : Step  Time=0  After=10  SampleTime=0
  Sum1 : Sum  Inputs=+++
  Sum4 : Sum  Inputs=|+-
  Sum5 : Sum  Inputs=|-+
  Sum57 : Sum  Inputs=++|
  Sum62 : Sum  Inputs=+++
  Transfer Fcn3 : TransferFcn  Numerator=[352535.4655]  Denominator=[1 59.56 2119 1.854e04]
  Erro PID : Outport
  Saída PID : Outport  Port=2
  Entrada PID : Outport  Port=3
  wires:
  Transfer Fcn3/1 -> Saída PID/1, Sum5/1, Sum4/2
  Sum1/1 -> Sum57/2
  Sum62/1 -> Sum5/2, Entrada PID/1, Sum4/1
  Gain2/1 -> Integrator2/1
  Gain1/1 -> Sum1/1
  Sum4/1 -> Gain1/1, Gain6/1, Gain2/1
  Gain6/1 -> Derivative2/1
  Step14/1 -> Sum62/2
  Step3/1 -> Sum62/1
  Step13/1 -> Sum62/3
  Step12/1 -> Sum57/1
  Derivative2/1 -> Sum1/3
  Sum57/1 -> Transfer Fcn3/1
  Integrator2/1 -> Sum1/2
  Sum5/1 -> Erro PID/1

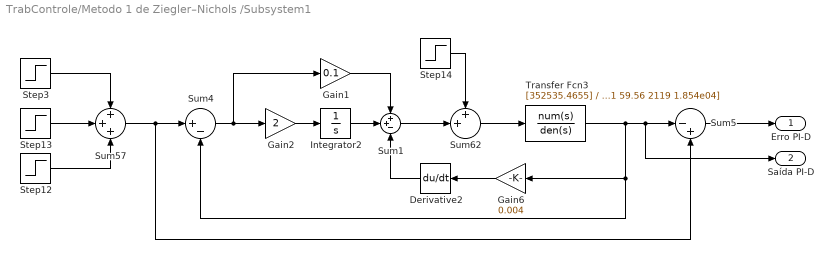
== system TrabControle/Metodo 1 de Ziegler–Nichols /Subsystem1 ==
  Derivative2 : Derivative
  Gain1 : Gain  Gain=0.1
  Gain2 : Gain  Gain=2
  Gain6 : Gain  Gain=0.004
  Integrator2 : Integrator
  Step12 : Step  Time=6  After=5  SampleTime=0
  Step13 : Step  Time=3  After=-10  SampleTime=0
  Step14 : Step  Time=8  After=2  SampleTime=0
  Step3 : Step  Time=0  After=10  SampleTime=0
  Sum1 : Sum  Inputs=++-
  Sum4 : Sum  Inputs=|+-
  Sum5 : Sum  Inputs=|-+
  Sum57 : Sum  Inputs=+++
  Sum62 : Sum  Inputs=++|
  Transfer Fcn3 : TransferFcn  Numerator=[352535.4655]  Denominator=[1 59.56 2119 1.854e04]
  Erro PI-D : Outport
  Saída PI-D : Outport  Port=2
  wires:
  Step13/1 -> Sum57/2
  Gain1/1 -> Sum1/1
  Derivative2/1 -> Sum1/3
  Sum4/1 -> Gain2/1, Gain1/1
  Integrator2/1 -> Sum1/2
  Transfer Fcn3/1 -> Sum4/2, Gain6/1, Saída PI-D/1, Sum5/1
  Sum5/1 -> Erro PI-D/1
  Sum1/1 -> Sum62/2
  Sum57/1 -> Sum5/2, Sum4/1
  Gain2/1 -> Integrator2/1
  Gain6/1 -> Derivative2/1
  Step12/1 -> Sum57/3
  Step14/1 -> Sum62/1
  Step3/1 -> Sum57/1
  Sum62/1 -> Transfer Fcn3/1

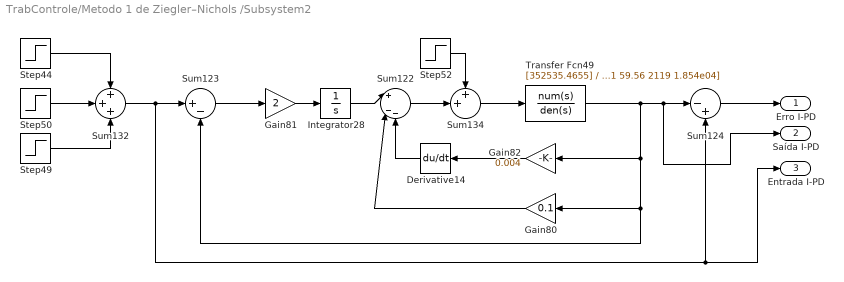
== system TrabControle/Metodo 1 de Ziegler–Nichols /Subsystem2 ==
  Derivative14 : Derivative
  Gain80 : Gain  Gain=0.1
  Gain81 : Gain  Gain=2
  Gain82 : Gain  Gain=0.004
  Integrator28 : Integrator
  Step44 : Step  Time=0  After=10  SampleTime=0
  Step49 : Step  Time=6  After=5  SampleTime=0
  Step50 : Step  Time=3  After=-10  SampleTime=0
  Step52 : Step  Time=8  After=2  SampleTime=0
  Sum122 : Sum  Inputs=|+|--
  Sum123 : Sum  Inputs=|+-
  Sum124 : Sum  Inputs=|-+
  Sum132 : Sum  Inputs=+++
  Sum134 : Sum  Inputs=++|
  Transfer Fcn49 : TransferFcn  Numerator=[352535.4655]  Denominator=[1 59.56 2119 1.854e04]
  Erro I-PD : Outport
  Saída I-PD : Outport  Port=2
  Entrada I-PD : Outport  Port=3
  wires:
  Step44/1 -> Sum132/1
  Sum132/1 -> Entrada I-PD/1, Sum124/2, Sum123/1
  Sum122/1 -> Sum134/2
  Sum123/1 -> Gain81/1
  Integrator28/1 -> Sum122/1
  Step52/1 -> Sum134/1
  Step50/1 -> Sum132/2
  Derivative14/1 -> Sum122/3
  Gain80/1 -> Sum122/2
  Transfer Fcn49/1 -> Sum123/2, Gain80/1, Gain82/1, Saída I-PD/1, Sum124/1
  Gain81/1 -> Integrator28/1
  Sum124/1 -> Erro I-PD/1
  Sum134/1 -> Transfer Fcn49/1
  Gain82/1 -> Derivative14/1
  Step49/1 -> Sum132/3

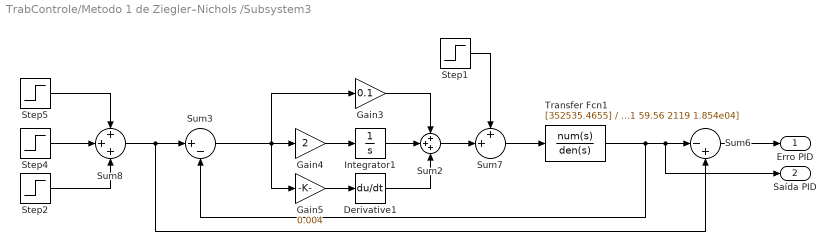
== system TrabControle/Metodo 1 de Ziegler–Nichols /Subsystem3 ==
  Derivative1 : Derivative
  Gain3 : Gain  Gain=0.1
  Gain4 : Gain  Gain=2
  Gain5 : Gain  Gain=0.004
  Integrator1 : Integrator
  Step1 : Step  Time=8  After=2  SampleTime=0
  Step2 : Step  Time=6  After=5  SampleTime=0
  Step4 : Step  Time=3  After=-10  SampleTime=0
  Step5 : Step  Time=0  After=10  SampleTime=0
  Sum2 : Sum  Inputs=+++
  Sum3 : Sum  Inputs=|+-
  Sum6 : Sum  Inputs=|-+
  Sum7 : Sum  Inputs=++|
  Sum8 : Sum  Inputs=+++
  Transfer Fcn1 : TransferFcn  Numerator=[352535.4655]  Denominator=[1 59.56 2119 1.854e04]
  Erro PID : Outport
  Saída PID : Outport  Port=2
  wires:
  Step2/1 -> Sum8/3
  Sum7/1 -> Transfer Fcn1/1
  Step1/1 -> Sum7/1
  Gain4/1 -> Integrator1/1
  Sum2/1 -> Sum7/2
  Integrator1/1 -> Sum2/2
  Derivative1/1 -> Sum2/3
  Sum6/1 -> Erro PID/1
  Step4/1 -> Sum8/2
  Sum8/1 -> Sum6/2, Sum3/1
  Gain3/1 -> Sum2/1
  Sum3/1 -> Gain3/1, Gain5/1, Gain4/1
  Transfer Fcn1/1 -> Saída PID/1, Sum6/1, Sum3/2
  Step5/1 -> Sum8/1
  Gain5/1 -> Derivative1/1

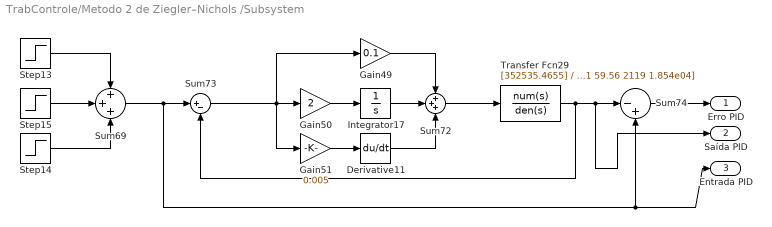
== system TrabControle/Metodo 2 de Ziegler–Nichols /Subsystem ==
  Derivative11 : Derivative
  Gain49 : Gain  Gain=0.1
  Gain50 : Gain  Gain=2
  Gain51 : Gain  Gain=0.005
  Integrator17 : Integrator
  Step13 : Step  Time=0  After=10  SampleTime=0
  Step14 : Step  Time=6  After=5  SampleTime=0
  Step15 : Step  Time=3  After=-10  SampleTime=0
  Sum69 : Sum  Inputs=+++
  Sum72 : Sum  Inputs=+++
  Sum73 : Sum  Inputs=|+-
  Sum74 : Sum  Inputs=|-+
  Transfer Fcn29 : TransferFcn  Numerator=[352535.4655]  Denominator=[1 59.56 2119 1.854e04]
  Erro PID : Outport
  Saída PID : Outport  Port=2
  Entrada PID : Outport  Port=3
  wires:
  Sum74/1 -> Erro PID/1
  Step14/1 -> Sum69/3
  Gain49/1 -> Sum72/1
  Sum73/1 -> Gain49/1, Gain51/1, Gain50/1
  Sum72/1 -> Transfer Fcn29/1
  Gain50/1 -> Integrator17/1
  Step15/1 -> Sum69/2
  Derivative11/1 -> Sum72/3
  Transfer Fcn29/1 -> Saída PID/1, Sum74/1, Sum73/2
  Sum69/1 -> Entrada PID/1, Sum74/2, Sum73/1
  Gain51/1 -> Derivative11/1
  Step13/1 -> Sum69/1
  Integrator17/1 -> Sum72/2

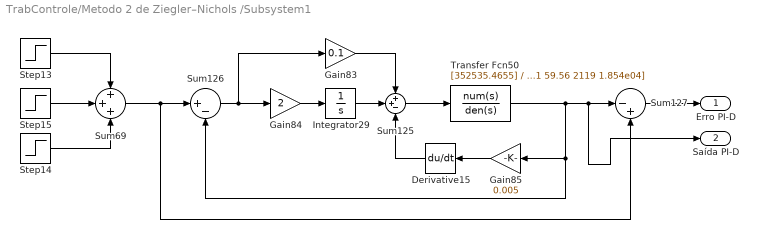
== system TrabControle/Metodo 2 de Ziegler–Nichols /Subsystem1 ==
  Derivative15 : Derivative
  Gain83 : Gain  Gain=0.1
  Gain84 : Gain  Gain=2
  Gain85 : Gain  Gain=0.005
  Integrator29 : Integrator
  Step13 : Step  Time=0  After=10  SampleTime=0
  Step14 : Step  Time=6  After=5  SampleTime=0
  Step15 : Step  Time=3  After=-10  SampleTime=0
  Sum125 : Sum  Inputs=++-
  Sum126 : Sum  Inputs=|+-
  Sum127 : Sum  Inputs=|-+
  Sum69 : Sum  Inputs=+++
  Transfer Fcn50 : TransferFcn  Numerator=[352535.4655]  Denominator=[1 59.56 2119 1.854e04]
  Erro PI-D : Outport
  Saída PI-D : Outport  Port=2
  wires:
  Sum127/1 -> Erro PI-D/1
  Sum126/1 -> Gain84/1, Gain83/1
  Gain85/1 -> Derivative15/1
  Gain83/1 -> Sum125/1
  Transfer Fcn50/1 -> Sum126/2, Gain85/1, Saída PI-D/1, Sum127/1
  Integrator29/1 -> Sum125/2
  Derivative15/1 -> Sum125/3
  Gain84/1 -> Integrator29/1
  Sum125/1 -> Transfer Fcn50/1
  Sum69/1 -> Sum127/2, Sum126/1
  Step15/1 -> Sum69/2
  Step13/1 -> Sum69/1
  Step14/1 -> Sum69/3

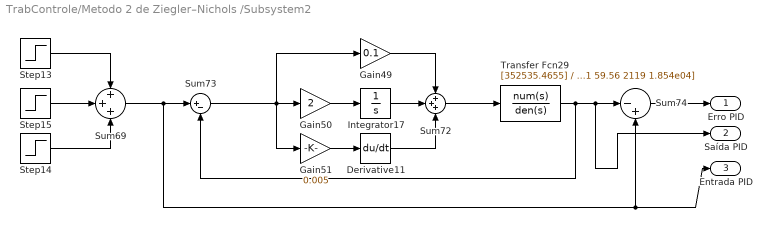
== system TrabControle/Metodo 2 de Ziegler–Nichols /Subsystem2 ==
  Derivative11 : Derivative
  Gain49 : Gain  Gain=0.1
  Gain50 : Gain  Gain=2
  Gain51 : Gain  Gain=0.005
  Integrator17 : Integrator
  Step13 : Step  Time=0  After=10  SampleTime=0
  Step14 : Step  Time=6  After=5  SampleTime=0
  Step15 : Step  Time=3  After=-10  SampleTime=0
  Sum69 : Sum  Inputs=+++
  Sum72 : Sum  Inputs=+++
  Sum73 : Sum  Inputs=|+-
  Sum74 : Sum  Inputs=|-+
  Transfer Fcn29 : TransferFcn  Numerator=[352535.4655]  Denominator=[1 59.56 2119 1.854e04]
  Erro PID : Outport
  Saída PID : Outport  Port=2
  Entrada PID : Outport  Port=3
  wires:
  Sum74/1 -> Erro PID/1
  Step14/1 -> Sum69/3
  Gain49/1 -> Sum72/1
  Sum73/1 -> Gain49/1, Gain51/1, Gain50/1
  Sum72/1 -> Transfer Fcn29/1
  Gain50/1 -> Integrator17/1
  Step15/1 -> Sum69/2
  Derivative11/1 -> Sum72/3
  Transfer Fcn29/1 -> Saída PID/1, Sum74/1, Sum73/2
  Sum69/1 -> Entrada PID/1, Sum74/2, Sum73/1
  Gain51/1 -> Derivative11/1
  Step13/1 -> Sum69/1
  Integrator17/1 -> Sum72/2

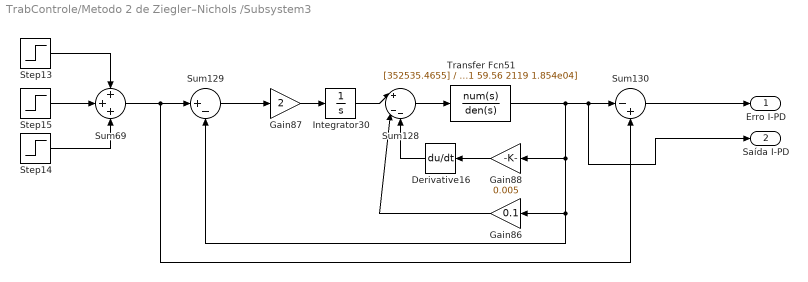
== system TrabControle/Metodo 2 de Ziegler–Nichols /Subsystem3 ==
  Derivative16 : Derivative
  Gain86 : Gain  Gain=0.1
  Gain87 : Gain  Gain=2
  Gain88 : Gain  Gain=0.005
  Integrator30 : Integrator
  Step13 : Step  Time=0  After=10  SampleTime=0
  Step14 : Step  Time=6  After=5  SampleTime=0
  Step15 : Step  Time=3  After=-10  SampleTime=0
  Sum128 : Sum  Inputs=|+|--
  Sum129 : Sum  Inputs=|+-
  Sum130 : Sum  Inputs=|-+
  Sum69 : Sum  Inputs=+++
  Transfer Fcn51 : TransferFcn  Numerator=[352535.4655]  Denominator=[1 59.56 2119 1.854e04]
  Erro I-PD : Outport
  Saída I-PD : Outport  Port=2
  wires:
  Sum130/1 -> Erro I-PD/1
  Derivative16/1 -> Sum128/3
  Sum129/1 -> Gain87/1
  Gain88/1 -> Derivative16/1
  Gain87/1 -> Integrator30/1
  Sum128/1 -> Transfer Fcn51/1
  Integrator30/1 -> Sum128/1
  Sum69/1 -> Sum130/2, Sum129/1
  Gain86/1 -> Sum128/2
  Transfer Fcn51/1 -> Sum129/2, Gain86/1, Gain88/1, Saída I-PD/1, Sum130/1
  Step15/1 -> Sum69/2
  Step13/1 -> Sum69/1
  Step14/1 -> Sum69/3
